simulink model "Questao_5"  (R2023b)
settings: Solver=VariableStepAuto  StartTime=0.0  StopTime=100  RelTol=1e-3
values from neighbouring files (symbols this model uses):
  B = 0.1    [setup.m]
  Kw = 1/3    (= 0.333333333333)    [setup.m]
  Ts = 0.162    [setup.m]
undefined symbols (not defined in the file or in its folder): DiscIntNeverNeededParam
settings Model: Creator=pedro  LastModifiedBy=pedro

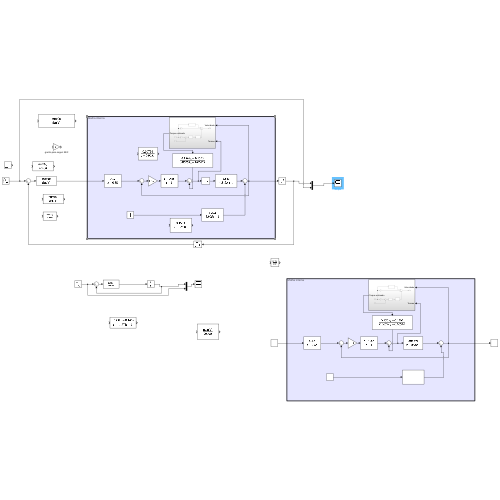
[thumbnail: Simulink's stored preview of the top-level diagram]
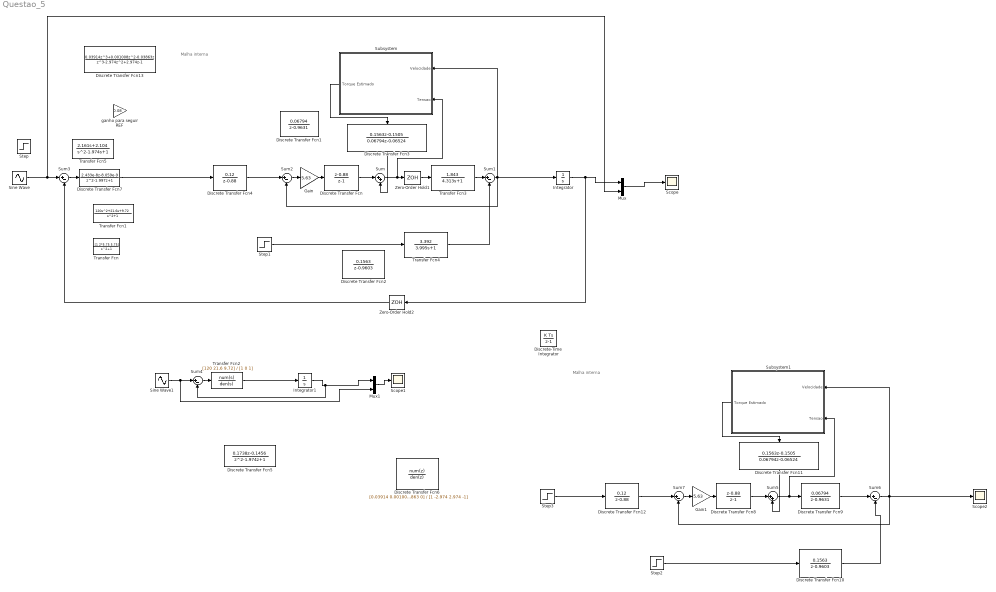
== system Questao_5 ==
  note: Malha interna
  note: Malha interna
  Discrete Transfer Fcn : DiscreteTransferFcn  Numerator=[1 -0.88]  Denominator=[1 -1]
  Discrete Transfer Fcn1 : DiscreteTransferFcn  Numerator=[0.06794]  Denominator=[1 -0.9631]
  Discrete Transfer Fcn10 : DiscreteTransferFcn  Numerator=[0.1563]  Denominator=[1 -0.9603]
  Discrete Transfer Fcn11 : DiscreteTransferFcn  Numerator=[0.1563 -0.1505]  Denominator=[0.06794 -0.06524]
  Discrete Transfer Fcn12 : DiscreteTransferFcn  Numerator=[0.12]  Denominator=[1 -0.88]
  Discrete Transfer Fcn13 : DiscreteTransferFcn  Numerator=[0.03914 0.001008 -0.03863 0]  Denominator=[1 -2.974 2.974 -1]
  Discrete Transfer Fcn2 : DiscreteTransferFcn  Numerator=[0.1563]  Denominator=[1 -0.9603]
  Discrete Transfer Fcn3 : DiscreteTransferFcn  Numerator=[0.1563 -0.1505]  Denominator=[0.06794 -0.06524]
  Discrete Transfer Fcn4 : DiscreteTransferFcn  Numerator=[0.12]  Denominator=[1 -0.88]
  Discrete Transfer Fcn5 : DiscreteTransferFcn  Numerator=[0.1738 -0.1456]  Denominator=[1 -1.974 1]
  Discrete Transfer Fcn6 : DiscreteTransferFcn  Numerator=[0.03914 0.001008 -0.03863 0]  Denominator=[1 -2.974 2.974 -1]
  Discrete Transfer Fcn7 : DiscreteTransferFcn  Numerator=[2.433e-8 -8.059e-9]  Denominator=[1 -1.997 1]
  Discrete Transfer Fcn8 : DiscreteTransferFcn  Numerator=[1 -0.88]  Denominator=[1 -1]
  Discrete Transfer Fcn9 : DiscreteTransferFcn  Numerator=[0.06794]  Denominator=[1 -0.9631]
  Discrete-Time Integrator : DiscreteIntegrator  SampleTime=0.162  UpperSaturationLimit=5  LowerSaturationLimit=-5  ICPrevOutput=DiscIntNeverNeededParam  ICPrevScaledInput=DiscIntNeverNeededParam
  Gain : Gain  Gain=5.63
  Gain1 : Gain  Gain=5.63
  Integrator : Integrator  LimitOutput=on  UpperSaturationLimit=5  LowerSaturationLimit=-5
  Integrator1 : Integrator  UpperSaturationLimit=5  LowerSaturationLimit=-5
  Mux : Mux  Inputs=2
  Mux1 : Mux  Inputs=2
  Scope : Scope
  Scope1 : Scope
  Scope2 : Scope
  Sine Wave : Sin  Frequency=0.1  SampleTime=0.162
  Sine Wave1 : Sin  SampleTime=0
  Step : Step  SampleTime=0.162
  Step1 : Step  Time=60  SampleTime=0.162
  Step2 : Step  Time=10  SampleTime=0.162
  Step3 : Step  SampleTime=0.162
  Subsystem : Subsystem
      settings: PortSchema="{\"entries\":[{\"content\":{\"sides\":[{\"content\":{},\"type\":\"ConnectorPlacement.EquallySpacedRectSide\",\"uuid\":\"e59a06e1-eab4-4bd2-85d9-68e257427de7\"},{\"content\":{\"side\":\"RIGHT\"},\"type\":\"ConnectorPlacement.EquallySpacedRectSide\",\"uuid\":\"6892985a-c8d8-4c3b-9c0c-3e543d6e16eb\"},{\"content\":{\"connectorIds\":[\"Out1\"],\"side\":\"TOP\"},\"type\":\"ConnectorPlacement.EquallySpacedRectSide\",\"uuid\":\"71dba93a-139c-4e39-b2a6-d594bacb8791\"},{\"content\":{\"connectorIds\":[\"In1\",\"In2\"],\"side\":\"BOTTOM\"},\"type\":\"ConnectorPlacement.EquallySpacedRectSide\",\"uuid\":\"1da54c87-6e6c-45c2-97e0-448bf39b9223\"}]},\"type\":\"ConnectorPlacement.EquallySpacedConnector\",\"uuid\":\"3219126c-845c-4a92-9507-56dbcc4fd8de\"}],\"packageUris\":[\"http://schema.mathworks.com/mf0/Connector/R2020b\"],\"version\":\"1.0\"}"
  Subsystem1 : Subsystem
      settings: PortSchema="{\"entries\":[{\"content\":{\"sides\":[{\"content\":{},\"type\":\"ConnectorPlacement.EquallySpacedRectSide\",\"uuid\":\"e59a06e1-eab4-4bd2-85d9-68e257427de7\"},{\"content\":{\"side\":\"RIGHT\"},\"type\":\"ConnectorPlacement.EquallySpacedRectSide\",\"uuid\":\"6892985a-c8d8-4c3b-9c0c-3e543d6e16eb\"},{\"content\":{\"connectorIds\":[\"Out1\"],\"side\":\"TOP\"},\"type\":\"ConnectorPlacement.EquallySpacedRectSide\",\"uuid\":\"71dba93a-139c-4e39-b2a6-d594bacb8791\"},{\"content\":{\"connectorIds\":[\"In1\",\"In2\"],\"side\":\"BOTTOM\"},\"type\":\"ConnectorPlacement.EquallySpacedRectSide\",\"uuid\":\"1da54c87-6e6c-45c2-97e0-448bf39b9223\"}]},\"type\":\"ConnectorPlacement.EquallySpacedConnector\",\"uuid\":\"3219126c-845c-4a92-9507-56dbcc4fd8de\"}],\"packageUris\":[\"http://schema.mathworks.com/mf0/Connector/R2020b\"],\"version\":\"1.0\"}"
  Sum : Sum  Inputs=|++
  Sum{1..4,6..7} (6 alike) : Sum  Inputs=|+-
  Sum5 : Sum  Inputs=|++
  Transfer Fcn : TransferFcn  Numerator=[1 2*5.75 5.75]  Denominator=[1 0 1]
  Transfer Fcn1 : TransferFcn  Numerator=[120 21.6 9.72]  Denominator=[1 0 1]
  Transfer Fcn2 : TransferFcn  Numerator=[120 21.6 9.72]  Denominator=[1 0 1]
  Transfer Fcn3 : TransferFcn  Numerator=[1.843]  Denominator=[4.313 1]
  Transfer Fcn4 : TransferFcn  Numerator=[3.392]  Denominator=[3.995 1]
  Transfer Fcn5 : TransferFcn  Numerator=[2.161 2.104]  Denominator=[1 -1.974 1]
  Zero-Order Hold1 : ZeroOrderHold  SampleTime=0.162
  Zero-Order Hold2 : ZeroOrderHold  SampleTime=1.62
  ganho para seguir REF : Gain  Gain=0.08
  wires:
  Discrete Transfer Fcn/1 -> Sum/1
  Discrete Transfer Fcn4/1 -> Sum2/1
  Step1/1 -> Transfer Fcn4/1
  Subsystem/1(Torque Estimado) -> Discrete Transfer Fcn3/1
  Sum/1 -> Zero-Order Hold1/1, Subsystem/2(Tensao)
  Sum2/1 -> Gain/1
  Gain/1 -> Discrete Transfer Fcn/1
  Mux/1 -> Scope/1
  Sum1/1 -> Integrator/1, Subsystem/1(Velocidade), Sum2/2
  Sine Wave/1 -> Mux/2, Sum3/1
  Sum4/1 -> Transfer Fcn2/1
  Mux1/1 -> Scope1/1
  Transfer Fcn4/1 -> Sum1/2
  Discrete Transfer Fcn3/1 -> Sum/2
  Sine Wave1/1 -> Mux1/2, Sum4/1
  Discrete Transfer Fcn7/1 -> Discrete Transfer Fcn4/1
  Sum5/1 -> Subsystem1/2(Tensao), Discrete Transfer Fcn9/1
  Sum6/1 -> Scope2/1, Subsystem1/1(Velocidade), Sum7/2
  Gain1/1 -> Discrete Transfer Fcn8/1
  Discrete Transfer Fcn8/1 -> Sum5/1
  Discrete Transfer Fcn9/1 -> Sum6/1
  Sum7/1 -> Gain1/1
  Subsystem1/1(Torque Estimado) -> Discrete Transfer Fcn11/1
  Step2/1 -> Discrete Transfer Fcn10/1
  Discrete Transfer Fcn10/1 -> Sum6/2
  Discrete Transfer Fcn12/1 -> Sum7/1
  Step3/1 -> Discrete Transfer Fcn12/1
  Discrete Transfer Fcn11/1 -> Sum5/2
  Integrator/1 -> Mux/1, Zero-Order Hold2/1
  Sum3/1 -> Discrete Transfer Fcn7/1
  Transfer Fcn2/1 -> Integrator1/1
  Integrator1/1 -> Mux1/1, Sum4/2
  Transfer Fcn3/1 -> Sum1/1
  Zero-Order Hold1/1 -> Transfer Fcn3/1
  Zero-Order Hold2/1 -> Sum3/2

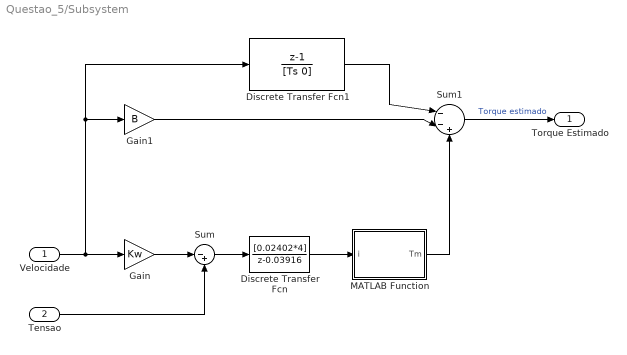
== system Questao_5/Subsystem ==
  Velocidade : Inport
  Tensao : Inport  Port=2
  Discrete Transfer Fcn : DiscreteTransferFcn  Numerator=[0.02402*4]  Denominator=[1 -0.03916]
  Discrete Transfer Fcn1 : DiscreteTransferFcn  Numerator=[1 -1]  Denominator=[Ts 0]
  Gain : Gain  Gain=Kw
  Gain1 : Gain  Gain=B
  MATLAB Function : MATLAB Function  TreatAsAtomicUnit=on
  Sum : Sum  Inputs=|-+
  Sum1 : Sum  Inputs=|--+
  Torque Estimado : Outport
  wires:
  Velocidade/1 -> Discrete Transfer Fcn1/1, Gain1/1, Gain/1
  Gain/1 -> Sum/1
  Tensao/1 -> Sum/2
  Sum/1 -> Discrete Transfer Fcn/1
  Discrete Transfer Fcn/1 -> MATLAB Function/1(i)
  MATLAB Function/1(Tm) -> Sum1/3
  Gain1/1 -> Sum1/2
  Discrete Transfer Fcn1/1 -> Sum1/1
  Sum1/1 -> Torque Estimado/1  "Torque estimado"

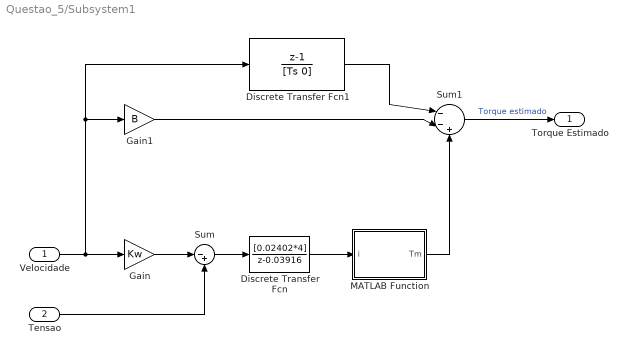
== system Questao_5/Subsystem1 ==
  Velocidade : Inport
  Tensao : Inport  Port=2
  Discrete Transfer Fcn : DiscreteTransferFcn  Numerator=[0.02402*4]  Denominator=[1 -0.03916]
  Discrete Transfer Fcn1 : DiscreteTransferFcn  Numerator=[1 -1]  Denominator=[Ts 0]
  Gain : Gain  Gain=Kw
  Gain1 : Gain  Gain=B
  MATLAB Function : MATLAB Function  TreatAsAtomicUnit=on
  Sum : Sum  Inputs=|-+
  Sum1 : Sum  Inputs=|--+
  Torque Estimado : Outport
  wires:
  Velocidade/1 -> Discrete Transfer Fcn1/1, Gain1/1, Gain/1
  Gain/1 -> Sum/1
  Tensao/1 -> Sum/2
  Sum/1 -> Discrete Transfer Fcn/1
  Discrete Transfer Fcn/1 -> MATLAB Function/1(i)
  MATLAB Function/1(Tm) -> Sum1/3
  Gain1/1 -> Sum1/2
  Discrete Transfer Fcn1/1 -> Sum1/1
  Sum1/1 -> Torque Estimado/1  "Torque estimado"

== matlab function Questao_5/Subsystem/MATLAB Function ==
  data: i input; Tm output
function Tm = fcn(i)

    if (i < 0)
        Tm = -5.26 * (1 - exp(i));

    else
        Tm = 5.26 * (1 - exp(-i));
    end

== matlab function Questao_5/Subsystem1/MATLAB Function ==
  data: i input; Tm output
function Tm = fcn(i)

    if (i < 0)
        Tm = -5.26 * (1 - exp(i));

    else
        Tm = 5.26 * (1 - exp(-i));
    end
